simulink model "variacion_K"  (R2026a)
settings: Solver=VariableStepAuto
values from neighbouring files (symbols this model uses):
  K = cambio_y / delta_u    [Taller_1_Identificacion_grafica_de_sistemas_FOTD.m]
  t_escalon = t(idx_escalon + 1)    [Taller_1_Identificacion_grafica_de_sistemas_FOTD.m]
  tau_analitico = 1.5 * (t_63_relativo - t_28_relativo)    [Taller_1_Identificacion_grafica_de_sistemas_FOTD.m]
  theta_analitico = t_63_relativo - tau_analitico    [Taller_1_Identificacion_grafica_de_sistemas_FOTD.m]
settings Model: Creator=Daniel  LastModifiedBy=Daniel

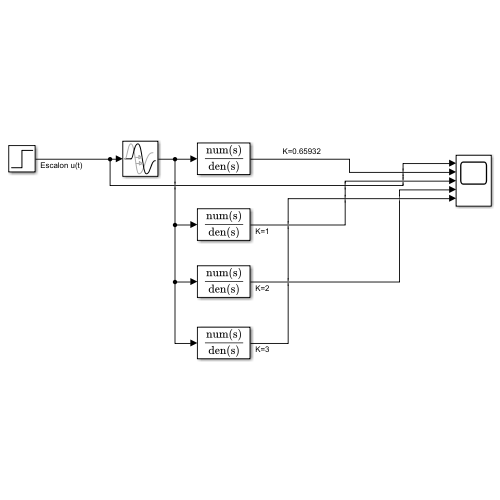
[thumbnail: Simulink's stored preview of the top-level diagram]
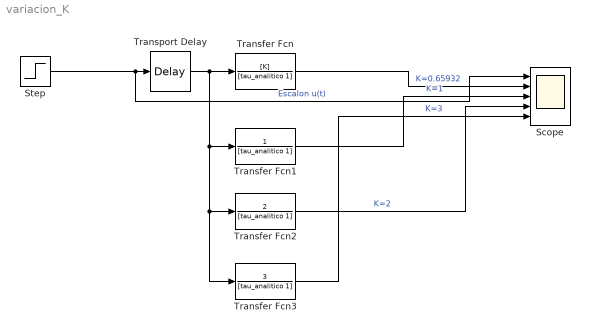
== system variacion_K ==
  Scope : Scope  NumInputPorts=5
      settings: Title=Respuesta del Modelo Analítico  ActiveDisplayYMinimum=-1.0234505837712371  ActiveDisplayYMaximum=4.5851858405649457  YLabel=Amplitud
  Step : Step  Time=t_escalon  FinalValue=1.5  SampleTime=0
  Transfer Fcn : TransferFcn  Numerator=[K]  Denominator=[tau_analitico 1]
  Transfer Fcn1 : TransferFcn  Denominator=[tau_analitico 1]
  Transfer Fcn2 : TransferFcn  Numerator=[2]  Denominator=[tau_analitico 1]
  Transfer Fcn3 : TransferFcn  Numerator=[3]  Denominator=[tau_analitico 1]
  Transport Delay : TransportDelay  DelayTime=theta_analitico
  wires:
  Transfer Fcn2/1 -> Scope/4  "K=2"
  Transfer Fcn1/1 -> Scope/3  "K=1"
  Transfer Fcn3/1 -> Scope/5  "K=3"
  Step/1 -> Scope/1, Transport Delay/1  "Escalon u(t)"
  Transfer Fcn/1 -> Scope/2  "K=0.65932"
  Transport Delay/1 -> Transfer Fcn3/1, Transfer Fcn2/1, Transfer Fcn1/1, Transfer Fcn/1
